simulink model "car_model"  (R2022b)
settings: Solver=VariableStepAuto  StartTime=0.0  StopTime=30  RelTol=1e-3
values from neighbouring files (symbols this model uses):
  X = Chassis_Signals.InertFrm.Cg.Disp.X.Data(:)    [Simulation_Data_Parse.m]    (also in Vehicle_Sim_Parse.m)
  Y = Chassis_Signals.InertFrm.Cg.Disp.Y.Data(:)    [Simulation_Data_Parse.m]    (also in Vehicle_Sim_Parse.m)
undefined symbols (not defined in the file or in its folder): ABS_MAX_TORQUE, ABS_MAX_TRQ_CMD, ABS_MIN_TORQUE, acc_IC, ACCELERATION_MAX, ActSuspDutyCycle, Aeq_left, Aeq_right, alpha_error, ang_acc_hystersesis, ang_IC, ang_vel_IC, area_air, axb, battery_current_IC, BATTERY_CURRENT_MAX, BATTERY_CURRENT_MIN, battery_FT_IC, battery_T_IC, BATTERY_TEMPERATURE_MAX, BATTERY_TEMPERATURE_MIN, battery_voltage_IC, BATTERY_VOLTAGE_MAX, BATTERY_VOLTAGE_MIN, Brake_Pressure_IC, ccl_IC, CENTER_STEER_ANGLE_MAX, covA, covarience_matrix_IC, covG, covM, covP, covV, cy_sweep, dB, dcl_IC, DCL_MAX, DCL_MIN, deadband_angle, dIndex, DiscIntNeverNeededParam, disk_abore, driver_t, dt_OFF, dt_ON, dTx, dx, dZ, F0z, forward_look_straight, forward_look_turn, fusion_t, fusion_t_sim, Fz_IC, Fz_sweep, g, gearbox_efficiency, gps_counter_IC, gps_ratio, gr ... (+105)
libraries: fl_lib x62, nesl_utility x16, vehdynlibtire x10, vehdynlibsuspension x8, simulink x5, autolibutils x5, sharedtransform x5, EngineCoolingComponents_lib x4, slpidlib x3, SimscapeFluids_lib x3, dspstat3 x2, shared6dof x2
(part 1 of 10)
settings Model: SimulationMode=accelerator  TunableVars=covA,covM,covP,covV,covG,phi,ref_location,ref_mag_field,location_lla_IC,gps_ratio,noise_state,fusion_t,ABS_MAX_TORQUE,MOTOR_ENABLE,BATTERY_CURRENT_MAX,deadband_angle,alpha_error,I,P,Torque_Up_Rate_Limit,Torque_Down_Rate_Limit,CURRENT_BUFFER,TVS_Intensity  TunableVarsStorageClass=Auto,Auto,Auto,Auto,Auto,Auto,Auto,Auto,Auto,Auto,Auto,Auto,Auto,Auto,Auto,Auto,Auto,Auto,Auto,Auto,Auto,Auto,Auto  TunableVarsTypeQualifier=,,,,,,,,,,,,,,,,,,,,,,  Creator=Inver  LastModifiedBy=Inver
settings DataIOCC: SaveFormat=StructureWithTime  SaveOutput=off  DSMLogging=off
settings OptimizationCC: DefaultParameterBehavior=Inlined  UseDivisionForNetSlopeComputation=on  GainParamInheritBuiltInType=on  UseFloatMulNetSlope=on  InlineInvariantSignals=on  PassReuseOutputArgsAs=Individual arguments  ZeroExternalMemoryAtStartup=off  ZeroInternalMemoryAtStartup=off  NoFixptDivByZeroProtection=on  EfficientFloat2IntCast=on  LifeSpan=1  OptimizeBlockOrder=speed  DifferentSizesBufferReuse=on  EfficientTunableParamExpr=on
settings DebuggingCC: ReadBeforeWriteMsg=DisableAll  WriteAfterWriteMsg=DisableAll  WriteAfterReadMsg=DisableAll  MultiTaskDSMMsg=none  ParameterTunabilityLossMsg=error  UnderSpecifiedDataTypeMsg=warning  UnderSpecifiedDimensionMsg=warning
settings HardwareCC: ProdBitPerPointer=32  ProdBitPerSizeT=32  ProdBitPerPtrDiffT=32  ProdLargestAtomicInteger=Long  ProdLargestAtomicFloat=Double  ProdWordSize=32  ProdLongLongMode=on  ProdHWDeviceType=ARM Compatible->ARM Cortex-M
settings ModelReferenceCC: EnableRefExpFcnMdlSchedulingChecks=on
settings SFSimCC: SimCustomHeaderCode="#include \"simplex.h\""  SimUserSources=C_Code/simplex.c  SFSimEcho=off  MATLABDynamicMemAlloc=off
settings RTWCC: Description=Embedded Coder  SystemTargetFile=ert.tlc  TemplateMakefile=ert_default_tmf  Toolchain=GNU Tools for ARM Embedded Processors
settings CodeAppCC: ForceParamTrailComments=on  IgnoreCustomStorageClasses=off  OperatorAnnotations=on  SimulinkDataObjDesc=on  SFDataObjDesc=on  CustomSymbolStrGlobalVar=rt$N$M  CustomSymbolStrType=$N$M  CustomSymbolStrFcn=$N$M$F  CustomSymbolStrMacro=$N$M  InsertBlockDesc=on
settings ERTTargetCC: TargetLangStandard=C99 (ISO)  GenerateSampleERTMain=on  IncludeMdlTerminateFcn=off  CombineSignalStateStructs=on  CodeInterfacePackaging=Reusable function  SupportComplex=off  SupportNonInlinedSFcns=on  InlinedParameterPlacement=NonHierarchical  RootIOFormat=Structure reference  ERTCustomFileTemplate=example_file_process.tlc  ERTFilePackagingFormat=CompactWithDataFile

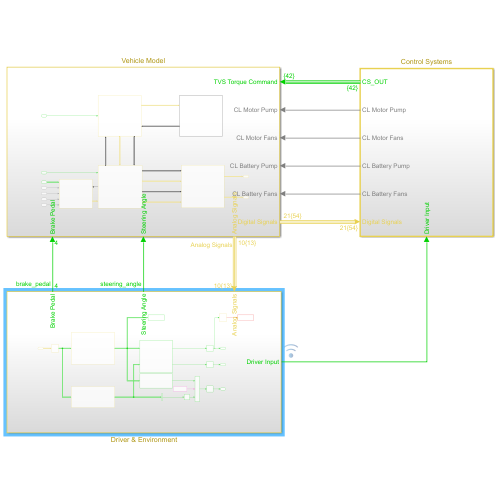
[thumbnail: Simulink's stored preview of the top-level diagram]
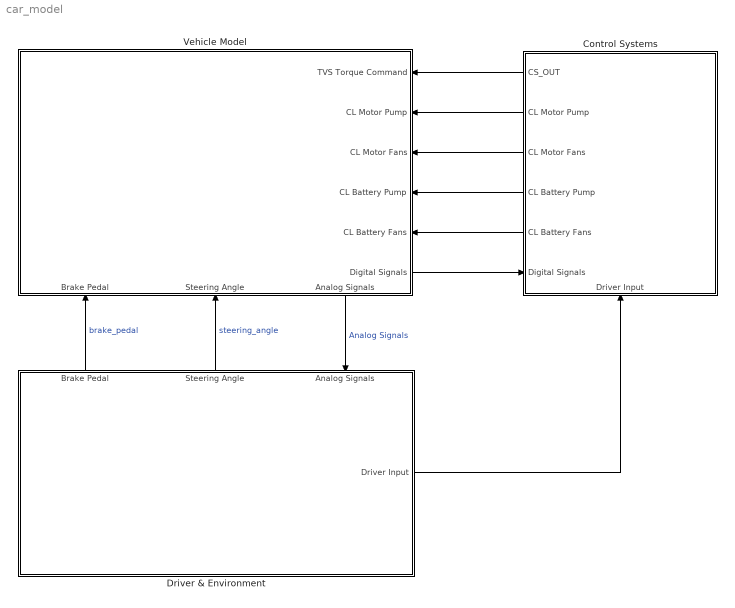
== system car_model ==
  Control Systems : Subsystem  TreatAsAtomicUnit=on  RTWFcnName=TVS_SYSTEM  RTWFileName=TVS_SYSTEM
      settings: PortSchema="{\"entries\":[{\"content\":{\"sides\":[{\"content\":{\"connectorIds\":[\"Out1\",\"Out2\",\"Out3\",\"Out4\",\"Out5\",\"In1\"]},\"type\":\"ConnectorPlacement.EquallySpacedRectSide\",\"uuid\":\"b5513b79-39cc-4156-8758-e9dd7d224c4f\"},{\"content\":{\"connectorIds\":[],\"side\":\"RIGHT\"},\"type\":\"ConnectorPlacement.EquallySpacedRectSide\",\"uuid\":\"18919d17-351d-4641-ab2c-66cbba916b4f\"},{\"content\":{\"connectorIds\":[],\"side\":\"TOP\"},\"type\":\"ConnectorPlacement.EquallySpacedRectSide\",\"uuid\":\"63240dfa-789e-427a-a529-4bce5e7f3f10\"},{\"content\":{\"connectorIds\":[\"In2\"],\"side\":\"BOTTOM\"},\"type\":\"ConnectorPlacement.EquallySpacedRectSide\",\"uuid\":\"43cc723f-5f4e-4e66-a14e-4ae2f3e16f9e\"}]},\"type\":\"ConnectorPlacement.EquallySpacedConnector\",\"uuid\":\"47be9ba7-cea3-4b3b-9ee6-e23e075e553b\"}],\"packageUris\":[\"http://schema.mathworks.com/mf0/Connector/R2020b\"],\"version\":\"1.0\"}"
  Driver & Environment : Subsystem
      settings: PortSchema="{\"entries\":[{\"content\":{\"sides\":[{\"content\":{\"connectorIds\":[]},\"type\":\"ConnectorPlacement.EquallySpacedRectSide\",\"uuid\":\"bd499254-800d-4f65-9d66-206e4f6126a9\"},{\"content\":{\"connectorIds\":[\"Out1\"],\"side\":\"RIGHT\"},\"type\":\"ConnectorPlacement.EquallySpacedRectSide\",\"uuid\":\"787bb70a-048d-46a8-9404-9c629bdce5fb\"},{\"content\":{\"connectorIds\":[\"Out2\",\"Out3\",\"In1\"],\"side\":\"TOP\"},\"type\":\"ConnectorPlacement.EquallySpacedRectSide\",\"uuid\":\"94a1f635-0878-46b0-949b-f2a3fa746134\"}]},\"type\":\"ConnectorPlacement.EquallySpacedConnector\",\"uuid\":\"f81a85a8-63b1-46ab-bae2-7f37115d6b57\"}],\"packageUris\":[\"http://schema.mathworks.com/mf0/Connector/R2020b\"],\"version\":\"1.0\"}"
  Vehicle Model : Subsystem
      settings: PortSchema="{\"entries\":[{\"content\":{\"sides\":[{\"content\":{\"connectorIds\":[]},\"type\":\"ConnectorPlacement.EquallySpacedRectSide\",\"uuid\":\"7263df3d-11c2-488e-998f-6bd776306b9c\"},{\"content\":{\"connectorIds\":[\"In3\",\"In4\",\"In5\",\"In6\",\"In7\",\"Out1\"],\"side\":\"RIGHT\"},\"type\":\"ConnectorPlacement.EquallySpacedRectSide\",\"uuid\":\"b0de89c2-35d2-4c59-81fc-f1f509ccf522\"},{\"content\":{\"connectorIds\":[],\"side\":\"TOP\"},\"type\":\"ConnectorPlacement.EquallySpacedRectSide\",\"uuid\":\"474ba072-8402-41d1-8015-97ca573757b9\"},{\"content\":{\"connectorIds\":[\"In1\",\"In2\",\"Out2\"],\"side\":\"BOTTOM\"},\"type\":\"ConnectorPlacement.EquallySpacedRectSide\",\"uuid\":\"2efad9e8-b0d8-4de5-bddc-0b63eaa22f81\"}]},\"type\":\"ConnectorPlacement.EquallySpacedConnector\",\"uuid\":\"426f55ca-7f3f-41f0-94e6-91e6d6304a5e\"}],\"packageUris\":[\"http://schema.mathworks.com/mf0/Connector/R2020b\"],\"version\":\"1.0\"}"
  wires:
  Control Systems/1(CS_OUT) -> Vehicle Model/3(TVS Torque Command)
  Driver & Environment/2(Brake Pedal) -> Vehicle Model/1(Brake Pedal)  "brake_pedal"
  Driver & Environment/3(Steering Angle) -> Vehicle Model/2(Steering Angle)  "steering_angle"
  Vehicle Model/2(Analog Signals) -> Driver & Environment/1(Analog Signals)  "Analog Signals"
  Vehicle Model/1(Digital Signals) -> Control Systems/1(Digital Signals)
  Driver & Environment/1(Driver Input) -> Control Systems/2(Driver Input)
  Control Systems/2(CL Motor Pump) -> Vehicle Model/4(CL Motor Pump)
  Control Systems/4(CL Battery Pump) -> Vehicle Model/6(CL Battery Pump)
  Control Systems/3(CL Motor Fans) -> Vehicle Model/5(CL Motor Fans)
  Control Systems/5(CL Battery Fans) -> Vehicle Model/7(CL Battery Fans)

== system car_model/Control Systems ==
  Digital Signals : Inport
  Driver Input : Inport  Port=2
  Bus Creator : BusCreator  Inputs=9
  Bus Selector : BusSelector  OutputSignals=Corner Dynamics Sensors.theta,Corner Dynamics Sensors.omega,Power Sensors.pwr_lmt,Power Sensors.motor_V,Power Sensors.motor_I,Power Sensors.batt_V,Power Sensors.batt_I,Cooling Sensors.motor_T,Cooling Sensors.mc_T
  Bus Selector1 : BusSelector  OutputSignals=Navigation Sensors.mag,Navigation Sensors.gyro,Navigation Sensors.acc,Navigation Sensors.pos,Navigation Sensors.vel
  Bus Selector2 : BusSelector  OutputSignals=angvel_VNED,vel_VNED
  Bus Selector3 : BusSelector  OutputSignals=Cooling Sensors.motor_T,Cooling Sensors.motor_FT,Cooling Sensors.batt_T,Cooling Sensors.batt_FT
  Bus Selector4 : BusSelector  OutputSignals=Corner Dynamics Sensors.shock_L,Corner Dynamics Sensors.FZ
  CLC : Subsystem
  NFE : Subsystem
  Sensor Fusion : Subsystem  TreatAsAtomicUnit=on  SystemSampleTime=fusion_t_sim
  TV Output Bus : BusCreator  Inputs=17
  TVS : Subsystem  TreatAsAtomicUnit=on  SystemSampleTime=tvs_t_sim
  To Workspace : ToWorkspace  VariableName=TV_Output  SaveFormat=Timeseries  SampleTime=-1
  To Workspace2 : ToWorkspace  VariableName=Sensor_Fused  SaveFormat=Timeseries  SampleTime=-1
  CS_OUT : Outport
  CL Motor Pump : Outport  Port=2
  CL Motor Fans : Outport  Port=3
  CL Battery Pump : Outport  Port=4
  CL Battery Fans : Outport  Port=5
  wires:
  Digital Signals/1 -> Bus Selector3/1, Bus Selector1/1, Bus Selector4/1, Bus Selector/1
  Bus Selector4/1 -> NFE/1(shock_L)  "<shock_L>"
  Bus Selector3/1 -> CLC/1(motor_temperature)  "<motor_T>"
  Bus Selector3/2 -> CLC/2(motor_fluid_temperature)  "<motor_FT>"
  Bus Selector3/3 -> CLC/3(battery_temperature)  "<batt_T>"
  Bus Selector3/4 -> CLC/4(battery_fluid_temperature)  "<batt_FT>"
  CLC/1(CL Motor Pump) -> CL Motor Pump/1
  CLC/2(CL Battery Pump) -> CL Battery Pump/1
  CLC/3(CL Motor Fans) -> CL Motor Fans/1
  CLC/4(CL Battery Fans) -> CL Battery Fans/1
  Bus Selector4/2 -> NFE/2(<Fz>)  "<FZ>"
  Bus Creator/1 -> To Workspace2/1, Bus Selector2/1
  Bus Selector1/1 -> Sensor Fusion/1(mag)  "<mag>"
  TV Output Bus/1 -> To Workspace/1, CS_OUT/1
  Driver Input/1 -> TVS/1(driver_input)
  NFE/1(Fz) -> TVS/11(Fz)
  Bus Selector2/1 -> TVS/12(angvel_VNED)  "<angvel_VNED>"
  Bus Selector1/2 -> Sensor Fusion/2(gyro)  "<gyro>"
  Bus Selector1/3 -> Sensor Fusion/3(accel)  "<acc>"
  Bus Selector1/4 -> Sensor Fusion/4(pos)  "<pos>"
  Bus Selector1/5 -> Sensor Fusion/5(vel)  "<vel>"
  Sensor Fusion/1(angvel_VNED) -> Bus Creator/1  "angvel_VNED"
  Sensor Fusion/2(ang_NED) -> Bus Creator/2  "ang_NED"
  Sensor Fusion/3(pos_VNED) -> Bus Creator/3  "pos_VNED"
  Sensor Fusion/4(vel_VNED) -> Bus Creator/4  "vel_VNED"
  Sensor Fusion/5(acc_VNED) -> Bus Creator/5  "acc_VNED"
  Sensor Fusion/6(mag_VNED) -> Bus Creator/6  "mag_VNED"
  Sensor Fusion/7(acc_bias_VNED) -> Bus Creator/7  "acc_bias_VNED"
  Sensor Fusion/8(gyro_bias_VNED) -> Bus Creator/8  "gyro_bias_VNED"
  Sensor Fusion/9(mag_bias_VNED) -> Bus Creator/9  "mag_bias_VNED"
  TVS/1(ref_yaw) -> TV Output Bus/1  "ref_yaw"
  TVS/2(beq) -> TV Output Bus/2  "beq"
  TVS/3(obj_gain) -> TV Output Bus/3  "obj_gain"
  TVS/4(lb) -> TV Output Bus/4  "lb"
  TVS/5(ub) -> TV Output Bus/5  "ub"
  TVS/6(windup) -> TV Output Bus/6  "windup"
  TVS/7(Aeq) -> TV Output Bus/7  "Aeq"
  TVS/8(b) -> TV Output Bus/8  "b"
  TVS/9(Tx) -> TV Output Bus/9  "Tx"
  TVS/10(bigM_flag) -> TV Output Bus/10  "bigM_flag"
  TVS/11(omega_m_TV) -> TV Output Bus/11  "omega_m"
  TVS/12(max_ang_acc) -> TV Output Bus/12  "max_ang_acc"
  TVS/13(min_ang_acc) -> TV Output Bus/13  "min_ang_acc"
  TVS/14(motor_I) -> TV Output Bus/14  "motor_I"
  TVS/15(motor_V) -> TV Output Bus/15  "motor_V"
  TVS/16(I_limits) -> TV Output Bus/16  "current_limits"
  TVS/17(batt_V) -> TV Output Bus/17  "battery_V"
  Bus Selector2/2 -> TVS/13(vel_VNED)  "<vel_VNED>"
  Bus Selector/1 -> TVS/2(steering_angle)  "<theta>"
  Bus Selector/2 -> TVS/3(omega)  "<omega>"
  Bus Selector/3 -> TVS/4(current_limits)  "<pwr_lmt>"
  Bus Selector/4 -> TVS/5(motor_voltage)  "<motor_V>"
  Bus Selector/5 -> TVS/6(motor_current)  "<motor_I>"
  Bus Selector/6 -> TVS/7(battery_voltage)  "<batt_V>"
  Bus Selector/7 -> TVS/8(battery_current)  "<batt_I>"
  Bus Selector/8 -> TVS/9(motor_temp)  "<motor_T>"
  Bus Selector/9 -> TVS/10(mc_temp)  "<mc_T>"

== system car_model/Driver & Environment ==
  Analog Signals : Inport
  Bus Selector : BusSelector  OutputSignals=Steering Angle
  Bus Selector1 : BusSelector  OutputSignals=GndFz
  Constant : Constant  Value=YAW_ENABLE
  Lateral Control : Subsystem
  Longitudinal Control : Subsystem
      settings: PortSchema="{\"entries\":[{\"content\":{\"sides\":[{\"content\":{\"connectorIds\":[\"In1\",\"In2\",\"In3\"]},\"type\":\"ConnectorPlacement.EquallySpacedRectSide\",\"uuid\":\"c84d1b45-47cb-44c3-9bb8-057964d890de\"},{\"content\":{\"connectorIds\":[\"Out1\",\"Out2\",\"In4\"],\"side\":\"RIGHT\"},\"type\":\"ConnectorPlacement.EquallySpacedRectSide\",\"uuid\":\"136455d0-d36a-4818-af11-72b5a1b8c27c\"},{\"content\":{\"connectorIds\":[],\"side\":\"TOP\"},\"type\":\"ConnectorPlacement.EquallySpacedRectSide\",\"uuid\":\"42b2ce8c-2720-4fbc-908c-f7068b304798\"}]},\"type\":\"ConnectorPlacement.EquallySpacedConnector\",\"uuid\":\"ec27d525-5c9d-4748-8b13-bb528198656f\"}],\"packageUris\":[\"http://schema.mathworks.com/mf0/Connector/R2020b\"],\"version\":\"1.0\"}"
  Rate Limiter : RateLimiter  RisingSlewLimit=MAX_DTHETA_DRIVER  FallingSlewLimit=-MAX_DTHETA_DRIVER  SampleTimeMode=inherited
  Rate Transition : RateTransition  OutPortSampleTime=driver_t
  Reference Generator : Subsystem
  Sweep Generator : Subsystem
  Switch : Switch  Criteria=u2 > Threshold  SaturateOnIntegerOverflow=off  InputSameDT=off
  To Workspace1 : ToWorkspace  VariableName=Throttle  SaveFormat=Timeseries  SampleTime=-1
  Unit Delay : UnitDelay  InitialCondition=Brake_Pressure_IC  SampleTime=driver_t  HasFrameUpgradeWarning=on
  Unit Delay1 : UnitDelay  SampleTime=driver_t  HasFrameUpgradeWarning=on
  Unit Delay2 : UnitDelay  SampleTime=driver_t  HasFrameUpgradeWarning=on
  Driver Input : Outport
  Brake Pedal : Outport  Port=2
  Steering Angle : Outport  Port=3
  wires:
  Longitudinal Control/2(brake_pedal) -> Unit Delay/1  "brake_pressure_pa"
  Lateral Control/1(steering_angle) -> Switch/1  "center_column_steering_angle_deg"
  Longitudinal Control/1(driver_input) -> Unit Delay2/1  "driver_input"
  Switch/1 -> Unit Delay1/1
  Analog Signals/1 -> Rate Transition/1
  Constant/1 -> Switch/2
  Rate Limiter/1 -> Switch/3
  Rate Transition/1 -> Bus Selector1/1, Sweep Generator/1(Analog Signals), Reference Generator/1(Analog Signals)
  Unit Delay1/1 -> Steering Angle/1, Longitudinal Control/4(In3)
  Unit Delay/1 -> Brake Pedal/1
  Reference Generator/1(Controller Information) -> Lateral Control/1(Controller Information), Longitudinal Control/1(Controller Information)
  Sweep Generator/1(Controller Information) -> Longitudinal Control/3(Sweep Information), Bus Selector/1
  Bus Selector/1 -> Rate Limiter/1  "<Steering Angle>"
  Unit Delay2/1 -> Driver Input/1, To Workspace1/1  "throttle"
  Bus Selector1/1 -> Longitudinal Control/2(In2)  "<GndFz>"

== system car_model/Vehicle Model ==
  Brake Pedal : Inport
  Steering Angle : Inport  Port=2
  TVS Torque Command : Inport  Port=3
  CL Motor Pump : Inport  Port=4
  CL Motor Fans : Inport  Port=5
  CL Battery Pump : Inport  Port=6
  CL Battery Fans : Inport  Port=7
  Electronics : Subsystem
  Powertrain : Subsystem
      settings: PortSchema="{\"entries\":[{\"content\":{\"sides\":[{\"content\":{\"connectorIds\":[\"In1\",\"In2\",\"In3\",\"In4\",\"In5\"]},\"type\":\"ConnectorPlacement.EquallySpacedRectSide\",\"uuid\":\"895a90fc-946f-4344-af69-c005acf2f614\"},{\"content\":{\"connectorIds\":[\"In6\",\"Out1\"],\"side\":\"RIGHT\"},\"type\":\"ConnectorPlacement.EquallySpacedRectSide\",\"uuid\":\"931fcb49-b75e-480c-a4d6-2f82b080d057\"},{\"content\":{\"connectorIds\":[],\"side\":\"TOP\"},\"type\":\"ConnectorPlacement.EquallySpacedRectSide\",\"uuid\":\"d1b12b51-387e-4553-b5da-149d57232505\"}]},\"type\":\"ConnectorPlacement.EquallySpacedConnector\",\"uuid\":\"0cb2c3dd-4627-421c-9ed4-7e8c572a9937\"}],\"packageUris\":[\"http://schema.mathworks.com/mf0/Connector/R2020b\"],\"version\":\"1.0\"}"
  Suspension : Subsystem  Variant=on  VariantControlMode=label  LabelModeActiveChoice=1
      settings: PortSchema="{\"entries\":[{\"content\":{\"sides\":[{\"content\":{\"connectorIds\":[\"In1\"]},\"type\":\"ConnectorPlacement.EquallySpacedRectSide\",\"uuid\":\"d90bf910-501d-4dd1-a367-d76bd42ab174\"},{\"content\":{\"connectorIds\":[\"Out1\",\"In3\"],\"side\":\"RIGHT\"},\"type\":\"ConnectorPlacement.EquallySpacedRectSide\",\"uuid\":\"1fe7da07-1086-4d5e-8baf-d5d069455d6e\"},{\"content\":{\"connectorIds\":[],\"side\":\"TOP\"},\"type\":\"ConnectorPlacement.EquallySpacedRectSide\",\"uuid\":\"6ff63b9e-45bb-47e9-90cd-47f8e0815e57\"},{\"content\":{\"connectorIds\":[\"In2\",\"Out2\",\"Out3\"],\"side\":\"BOTTOM\"},\"type\":\"ConnectorPlacement.EquallySpacedRectSide\",\"uuid\":\"116c6de0-7bfa-4dc1-bfd0-57a2fffb3aa0\"}]},\"type\":\"ConnectorPlacement.EquallySpacedConnector\",\"uuid\":\"6475b998-12b0-4b0e-8a20-c379b8e08c7c\"}],\"packageUris\":[\"http://schema.mathworks.com/mf0/Connector/R2020b\"],\"version\":\"1.0\"}"
      mask Display:
      | switch str2num(get_param(gcb,'ActiveVariant'))
      |     case 1
      |         image('suspdw.png');
      |     case 2
      |         image([imread('suspindmap.png');imread('suspsamap.png')]);
      |     case 3
      |          image([imread('suspmacp.png');imread('suspsacoil.png')]);
      |     case 4
      |          image('suspmacp.png');
      |     case 5
      |          image('suspindmap.png');
      |     case 6
      |          image('suspkandc.png');
      | end
  Vehicle : Subsystem
      settings: PortSchema="{\"entries\":[{\"content\":{\"sides\":[{\"content\":{\"connectorIds\":[\"In1\",\"Out1\"]},\"type\":\"ConnectorPlacement.EquallySpacedRectSide\",\"uuid\":\"63fa377f-0583-4c60-bac7-9bd73dadd9a1\"},{\"content\":{\"connectorIds\":[],\"side\":\"RIGHT\"},\"type\":\"ConnectorPlacement.EquallySpacedRectSide\",\"uuid\":\"7f668e34-aa5e-4f2f-9be8-80fbb83ff2c8\"},{\"content\":{\"connectorIds\":[],\"side\":\"TOP\"},\"type\":\"ConnectorPlacement.EquallySpacedRectSide\",\"uuid\":\"511f439c-568f-45f1-9ff4-54e644eb8180\"}]},\"type\":\"ConnectorPlacement.EquallySpacedConnector\",\"uuid\":\"b54bf87e-fa06-468b-8fa9-38148d60ed3d\"}],\"packageUris\":[\"http://schema.mathworks.com/mf0/Connector/R2020b\"],\"version\":\"1.0\"}"
      mask Display: image('6dofcar.png');
  Wheels and Tires : Subsystem
      settings: PortSchema="{\"entries\":[{\"content\":{\"sides\":[{\"content\":{\"connectorIds\":[\"In1\",\"Out6\",\"In2\"]},\"type\":\"ConnectorPlacement.EquallySpacedRectSide\",\"uuid\":\"77263124-783e-4307-b979-a6212540af24\"},{\"content\":{\"connectorIds\":[\"Out1\",\"Out2\",\"Out3\",\"Out4\"],\"side\":\"RIGHT\"},\"type\":\"ConnectorPlacement.EquallySpacedRectSide\",\"uuid\":\"cb03b446-69c2-4dbf-929b-d33818acfe8b\"},{\"content\":{\"connectorIds\":[\"Out5\",\"In3\",\"In4\"],\"side\":\"TOP\"},\"type\":\"ConnectorPlacement.EquallySpacedRectSide\",\"uuid\":\"8e7e4023-62e5-48a8-8666-b4c8bb14cd01\"}]},\"type\":\"ConnectorPlacement.EquallySpacedConnector\",\"uuid\":\"1061f0db-ec8e-49bd-8d66-b4a53eaeacfa\"}],\"packageUris\":[\"http://schema.mathworks.com/mf0/Connector/R2020b\"],\"version\":\"1.0\"}"
      mask Display: image('wheel3dof.png')
  Digital Signals : Outport  PortDimensions={292}
  Analog Signals : Outport  Port=2  PortDimensions={292}
  wires:
  Steering Angle/1 -> Suspension/1(Steering)
  Suspension/1(Suspension) -> Vehicle/1(Suspension)  "Susp"
  Wheels and Tires/5(Wheels2Susp) -> Suspension/2(Wheel)
  Powertrain/1(PwrTrn) -> Wheels and Tires/2(PwrTrn)
  Brake Pedal/1 -> Wheels and Tires/1(Brake Press)
  TVS Torque Command/1 -> Powertrain/1(TVS Torque Command)
  Suspension/2(Suspension1) -> Wheels and Tires/3(Sus)
  Vehicle/1(VehFdbk) -> Suspension/3(Vehicle)  "Vehicle"
  Suspension/3(Veh) -> Wheels and Tires/4(Veh)
  Wheels and Tires/1(Vehicle) -> Electronics/1(Veh)  "veh"
  Wheels and Tires/2(Suspension) -> Electronics/2(Sus)  "sus"
  Wheels and Tires/3(Wheels) -> Electronics/3(Whl)  "whl"
  Electronics/1(Analog Signals) -> Analog Signals/1
  Electronics/2(Digital Signals) -> Digital Signals/1
  Wheels and Tires/4(Power Train) -> Electronics/4(Trn)  "trn"
  CL Motor Pump/1 -> Powertrain/2(CL Motor Pump)
  CL Battery Pump/1 -> Powertrain/4(CL Battery Pump)
  CL Motor Fans/1 -> Powertrain/3(CL Motor Fans)
  CL Battery Fans/1 -> Powertrain/5(CL Battery Fans)
  Wheels and Tires/6(Vg) -> Powertrain/6(Vg)

== system car_model/Control Systems/CLC ==
  motor_temperature : Inport
  motor_fluid_temperature : Inport  Port=2
  battery_temperature : Inport  Port=3
  battery_fluid_temperature : Inport  Port=4
  Step : Step  After=0  SampleTime=0
  CL Motor Pump : Outport
  CL Battery Pump : Outport  Port=2
  CL Motor Fans : Outport  Port=3
  CL Battery Fans : Outport  Port=4
  wires:
  Step/1 -> CL Motor Fans/1, CL Battery Fans/1, CL Battery Pump/1, CL Motor Pump/1

== system car_model/Control Systems/NFE ==
  shock_L : Inport
  <Fz> : Inport  Port=2
  Saturation17 : Saturate  UpperLimit=1200  LowerLimit=200
  Terminator : Terminator
  Fz : Outport
  wires:
  shock_L/1 -> Terminator/1
  <Fz>/1 -> Saturation17/1
  Saturation17/1 -> Fz/1  "FZ"

== system car_model/Control Systems/Sensor Fusion ==
  mag : Inport
  gyro : Inport  Port=2
  accel : Inport  Port=3
  pos : Inport  Port=4
  vel : Inport  Port=5
  NED2VNED : MATLAB Function  TreatAsAtomicUnit=on
  SNED to VNED : MATLAB Function  TreatAsAtomicUnit=on
  Transpose{,1..11} (12 alike) : Math  Operator=transpose
  Unit Delay1 : UnitDelay  InitialCondition=gps_counter_IC  SampleTime=-1  HasFrameUpgradeWarning=on
  Unit Delay2 : UnitDelay  InitialCondition=state_IC  SampleTime=-1  HasFrameUpgradeWarning=on
  Unit Delay3 : UnitDelay  InitialCondition=covarience_matrix_IC  SampleTime=-1  HasFrameUpgradeWarning=on
  fusion : MATLAB Function  TreatAsAtomicUnit=on
  angvel_VNED : Outport
  ang_NED : Outport  Port=2
  pos_VNED : Outport  Port=3
  vel_VNED : Outport  Port=4
  acc_VNED : Outport  Port=5
  mag_VNED : Outport  Port=6
  acc_bias_VNED : Outport  Port=7
  gyro_bias_VNED : Outport  Port=8
  mag_bias_VNED : Outport  Port=9
  wires:
  NED2VNED/7(accel_bias) -> Transpose8/1  "acc_bias_VNED"
  NED2VNED/3(pos) -> Transpose9/1  "pos_VNED"
  NED2VNED/4(vel) -> Transpose5/1  "vel_VNED"
  NED2VNED/2(angvel) -> Transpose10/1  "angvel_VNED"
  NED2VNED/1(ang) -> Transpose11/1  "ang_NED"
  fusion/2(rot_map) -> NED2VNED/1(rot_map)
  Transpose/1 -> fusion/4(acceleration)
  Unit Delay3/1 -> fusion/8(cov_in)
  NED2VNED/8(gyro_bias) -> Transpose4/1  "gyro_bias_VNED"
  Transpose1/1 -> fusion/5(angularVelocity)
  fusion/4(cov_out) -> Unit Delay3/1
  fusion/3(state_out) -> Unit Delay2/1, NED2VNED/2(state)
  SNED to VNED/2(gyro_VNED) -> Transpose1/1  "gyro_VNED"
  SNED to VNED/1(accel_VNED) -> Transpose/1  "accel_VNED"
  NED2VNED/5(accel) -> Transpose6/1  "acc_VNED"
  SNED to VNED/3(mag_VNED) -> Transpose2/1  "mag_VNED"
  Unit Delay2/1 -> fusion/7(state_in)
  Transpose2/1 -> fusion/6(magField)
  NED2VNED/9(mag_bias) -> Transpose3/1  "mag_bias_VNED"
  NED2VNED/6(mag) -> Transpose7/1  "mag_VNED"
  accel/1 -> SNED to VNED/1(accel_SNED)
  gyro/1 -> SNED to VNED/2(gyro_SNED)
  mag/1 -> SNED to VNED/3(mag_SNED)
  pos/1 -> fusion/3(position)
  vel/1 -> fusion/2(velocity)
  Transpose3/1 -> mag_bias_VNED/1
  Transpose4/1 -> gyro_bias_VNED/1
  Transpose8/1 -> acc_bias_VNED/1
  Transpose7/1 -> mag_VNED/1
  Transpose6/1 -> acc_VNED/1
  Transpose5/1 -> vel_VNED/1
  Transpose9/1 -> pos_VNED/1
  Transpose10/1 -> angvel_VNED/1
  Transpose11/1 -> ang_NED/1
  fusion/1(count) -> Unit Delay1/1
  Unit Delay1/1 -> fusion/1("count ")

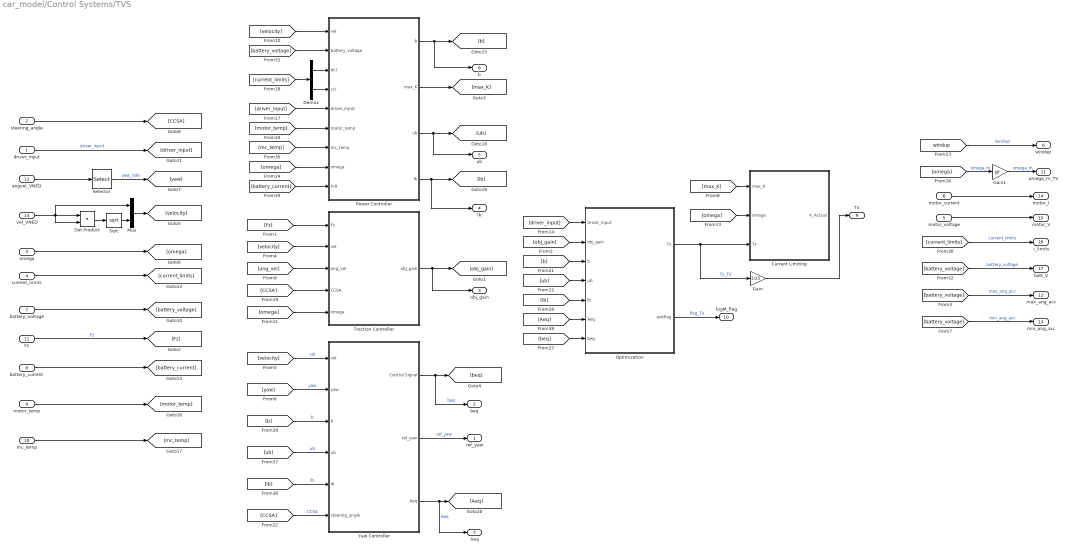
== system car_model/Control Systems/TVS ==
  driver_input : Inport  OutMin=-1  OutMax=1  OutDataTypeStr=double  PortDimensions=1  LockScale=on
  steering_angle : Inport  Port=2  OutMin=-130  OutMax=130  OutDataTypeStr=double  PortDimensions=1
  omega : Inport  Port=3  OutMin=0  OutMax=150  OutDataTypeStr=double  LockScale=on
  current_limits : Inport  Port=4  OutMin=-80000  OutMax=80000  OutDataTypeStr=double  LockScale=on
  motor_voltage : Inport  Port=5
  motor_current : Inport  Port=6
  battery_voltage : Inport  Port=7  OutMin=50  OutMax=340  OutDataTypeStr=double
  battery_current : Inport  Port=8
  motor_temp : Inport  Port=9
  mc_temp : Inport  Port=10
  Fz : Inport  Port=11
  angvel_VNED : Inport  Port=12  OutMin=-5  OutMax=5  OutDataTypeStr=double  PortDimensions=[1 3]  LockScale=on
  vel_VNED : Inport  Port=13  OutMin=0  OutMax=30  OutDataTypeStr=double  LockScale=on
  Current Limiting : Subsystem
  Demux : Demux  Outputs=2
  Dot Product : DotProduct  OutDataTypeStr=Inherit: Inherit via internal rule
  Gain : Gain  Gain=1/25
  Gain1 : Gain  Gain=gr  ParamDataTypeStr=double  OutDataTypeStr=Inherit: Inherit via back propagation
  Mux : Mux  Inputs=2
  Optimization : Subsystem
  Power Controller : Subsystem
  Selector : Selector  InputPortWidth=3  IndexOptions=Index vector (dialog)  Indices=3  OutputSizes=1
  Sqrt : Sqrt
  Traction Controller : Subsystem
  Yaw Controller : Subsystem
  ref_yaw : Outport
  beq : Outport  Port=2  OutMin=-10  OutMax=10  OutDataTypeStr=double  LockScale=on
  obj_gain : Outport  Port=3
  lb : Outport  Port=4  OutMin=-25  OutMax=25  OutDataTypeStr=double  LockScale=on
  ub : Outport  Port=5  OutMin=-25  OutMax=25  OutDataTypeStr=double  LockScale=on
  windup : Outport  Port=6
  Aeq : Outport  Port=7  OutMin=-1.9  OutMax=1.9  OutDataTypeStr=double  LockScale=on
  b : Outport  Port=8  OutMin=-80000  OutMax=80000  OutDataTypeStr=double  LockScale=on
  Tx : Outport  Port=9  OutDataTypeStr=double  PortDimensions=[1 4]
  bigM_flag : Outport  Port=10  PortDimensions=1
  omega_m_TV : Outport  Port=11
  max_ang_acc : Outport  Port=12
  min_ang_acc : Outport  Port=13
  motor_I : Outport  Port=14
  motor_V : Outport  Port=15
  I_limits : Outport  Port=16
  batt_V : Outport  Port=17
  wires:
  motor_current/1 -> motor_I/1
  motor_voltage/1 -> motor_V/1
  omega/1 -> [omega]
  [velocity] -> Traction Controller/2(vel)
  current_limits/1 -> [current_limits]
  Optimization/2(exitflag) -> bigM_flag/1  "flag_TV"
  vel_VNED/1 -> Mux/1, Dot Product/2, Dot Product/1
  [omega] -> Gain1/1  "omega_m"
  [velocity] -> Yaw Controller/1(vel)  "vel"
  [ang_vel] -> Traction Controller/3(ang_vel)
  Power Controller/1(b) -> b/1, [b]
  Traction Controller/1(obj_gain) -> [obj_gain], obj_gain/1
  Power Controller/3(ub) -> ub/1, [ub]
  angvel_VNED/1 -> Selector/1
  [omega] -> Traction Controller/5(omega)
  battery_voltage/1 -> [battery_voltage]
  [driver_input] -> Optimization/1(driver_input)
  Yaw Controller/1(Control Signal) -> [beq], beq/1  "beq"
  [yaw] -> Yaw Controller/2(yaw)  "yaw"
  [Fz] -> Traction Controller/1(Fz)
  [windup] -> windup/1  "windup"
  Yaw Controller/3(Aeq) -> [Aeq], Aeq/1  "Aeq"
  driver_input/1 -> [driver_input]  "driver_input"
  [beq] -> Optimization/7(beq)
  Power Controller/4(lb) -> lb/1, [lb]
  Fz/1 -> [Fz]  "Fz"
  [obj_gain] -> Optimization/2(obj_gain)
  Yaw Controller/2(ref_yaw) -> ref_yaw/1  "ref_yaw"
  [current_limits] -> I_limits/1  "current_limits"
  [battery_voltage] -> batt_V/1  "battery_voltage"
  battery_current/1 -> [battery_current]
  Selector/1 -> [yaw]  "yaw_rate"
  Dot Product/1 -> Sqrt/1
  Mux/1 -> [velocity]
  Sqrt/1 -> Mux/2
  motor_temp/1 -> [motor_temp]
  mc_temp/1 -> [mc_temp]
  Gain1/1 -> omega_m_TV/1  "omega_m"
  steering_angle/1 -> [CCSA]
  [CCSA] -> Traction Controller/4(CCSA)
  [velocity] -> Power Controller/1(vel)
  [battery_voltage] -> Power Controller/2(battery_voltage)
  [battery_current] -> Power Controller/9(In9)
  [driver_input] -> Power Controller/5(driver_input)
  [motor_temp] -> Power Controller/6(motor_temp)
  [mc_temp] -> Power Controller/7(mc_temp)
  [current_limits] -> Demux/1
  Demux/2 -> Power Controller/4(ccl)
  Demux/1 -> Power Controller/3(dcl)
  [CCSA] -> Yaw Controller/6(steering_angle)  "CCSA"
  [ub] -> Optimization/4(ub)
  [lb] -> Optimization/5(lb)
  [b] -> Optimization/3(b)
  [ub] -> Yaw Controller/4(ub)  "ub"
  [lb] -> Yaw Controller/5(lb)  "lb"
  [b] -> Yaw Controller/3(b)  "b"
  [Aeq] -> Optimization/6(Aeq)
  [omega] -> Power Controller/8(omega)
  [battery_voltage] -> max_ang_acc/1  "max_ang_acc"
  [battery_voltage] -> min_ang_acc/1  "min_ang_acc"
  [max_K] -> Current Limiting/1(max_K)
  Power Controller/2(max_K) -> [max_K]
  [omega] -> Current Limiting/2(omega)
  Optimization/1(Tx) -> Gain/1, Current Limiting/3(Tx)  "Tx_TV"
  Gain/1 -> Tx/1

== system car_model/Driver & Environment/Lateral Control ==
  Controller Information : Inport
  1-D Lookup Table : Lookup_n-D  NumberOfTableDimensions=1  BreakpointsForDimension1=velocity_sweep  Table=max_yaw  ExtrapMethod=Clip  InternalRulePriority=Speed  RndMeth=Simplest
  2-D Lookup Table1 : Lookup_n-D  BreakpointsForDimension1=yaw_rate_sweep  BreakpointsForDimension2=velocity_sweep  Table=steering_Up_Grid  ExtrapMethod=Clip  InternalRulePriority=Speed  RndMeth=Simplest
      settings: InputPortMap=u0,u1
  2-D Lookup Table2 : Lookup_n-D  BreakpointsForDimension1=yaw_rate_sweep  BreakpointsForDimension2=velocity_sweep  Table=steering_Up_Grid  ExtrapMethod=Clip  InternalRulePriority=Speed  RndMeth=Simplest
      settings: InputPortMap=u0,u1
  Abs : Abs  SaturateOnIntegerOverflow=off
  Bus Selector : BusSelector  OutputSignals=p_error,Vnow,yaw_ref,v_cog
  Constant : Constant  Value=17.5
  Constant1 : Constant  Value=0
  GreaterThan : RelationalOperator  Operator=>  OutDataTypeStr=boolean  RndMeth=Simplest  InputSameDT=off
  GreaterThan1 : RelationalOperator  Operator=~=  OutDataTypeStr=boolean  RndMeth=Simplest  InputSameDT=off
  Min : MinMax  Inputs=2
  NAND : Logic  Operator=NAND  IconShape=distinctive  AllPortsSameDT=off  OutDataTypeStr=boolean
  NOT : Logic  Operator=NOT  IconShape=distinctive  AllPortsSameDT=off  OutDataTypeStr=boolean
  PID Controller : slpidlib/PID Controller  Controller=PID  Form=Parallel  TimeDomain=Discrete-time  UseExternalTs=off  SampleTime=-1  IntegratorMethod=Forward Euler  FilterMethod=Forward Euler  ControllerParametersSource=internal  P=P_Straight_Adjust  I=0  UseKiTs=on  D=0  N=0  UseFilter=on  TunerSelectOption=Transfer Function Based (PID Tuner App)  InitialConditionSource=internal  InitialConditionForIntegrator=0  InitialConditionForFilter=0  DifferentiatorICPrevScaledInput=0  ExternalReset=none  TrackingMode=off  Kt=1  LimitOutput=on  SatLimitsSource=internal  UpperSaturationLimit=MAX_STEERING_ADJUST  LowerSaturationLimit=-MAX_STEERING_ADJUST  LinearizeAsGain=on  AntiWindupMode=none  Kb=1  LimitIntegrator=off  UpperIntegratorSaturationLimit=inf  LowerIntegratorSaturationLimit=-inf  POutMin=[]  POutMax=[]  IOutMin=[]  IOutMax=[]  DOutMin=[]  DOutMax=[]  NOutMin=[]  NOutMax=[]  SumOutMin=[]  SumOutMax=[]  SaturationOutMin=[]  SaturationOutMax=[]  PParamMin=[]  PParamMax=[]  IParamMin=[]  IParamMax=[]  DParamMin=[]  DParamMax=[]  NParamMin=[]  NParamMax=[]  KbParamMin=[]  KbParamMax=[]  KtParamMin=[]  KtParamMax=[]  KbOutMin=[]  KbOutMax=[]  KtOutMin=[]  KtOutMax=[]  IntegratorOutMin=[]  IntegratorOutMax=[]  FilterOutMin=[]  FilterOutMax=[]  SumI1OutMin=[]  SumI1OutMax=[]  SumI2OutMin=[]  SumI2OutMax=[]  SumI3OutMin=[]  SumI3OutMax=[]  SumI4OutMin=[]  SumI4OutMax=[]  SumDOutMin=[]  SumDOutMax=[]  DifferentiatorOutMin=[]  DifferentiatorOutMax=[]  FilterDiffOutCoefMin=[]  FilterDiffOutCoefMax=[]  ReciprocalOutMin=[]  ReciprocalOutMax=[]  SumDenOutMin=[]  SumDenOutMax=[]  SumNumOutMin=[]  SumNumOutMax=[]  DivideOutMin=[]  DivideOutMax=[]  UdiffTsProdOutMin=[]  UdiffTsProdOutMax=[]  NTsProdOutMin=[]  NTsProdOutMax=[]  UintegralTsProdOutMin=[]  UintegralTsProdOutMax=[]  UngainTsProdOutMin=[]  UngainTsProdOutMax=[]  ClampingZeroOutDataTypeStr=Inherit: Inherit via back propagation  ClampingZeroOutMin=[]  ClampingZeroOutMax=[]  FilterDenConstantOutDataTypeStr=Inherit: Inherit via back propagation  FilterDenConstantOutMin=[]  FilterDenConstantOutMax=[]  PCopyOutDataTypeStr=Inherit: Inherit via back propagation  PCopyOutMin=[]  PCopyOutMax=[]  NCopyOutDataTypeStr=Inherit: Inherit via back propagation  NCopyOutMin=[]  NCopyOutMax=[]  IntegratorContinuousStateAttributes=''  IntegratorStateMustResolveToSignalObject=off  IntegratorRTWStateStorageClass=Auto  FilterContinuousStateAttributes=''  FilterStateMustResolveToSignalObject=off  FilterRTWStateStorageClass=Auto  ParallelPVariant=InternalParameters  IdealPVariant=Disabled  IVariant=InternalParameters  DVariant=InternalParameters  IntegratorVariant=Discrete  SatVariant=Enabled  AWVariant=Passthrough  PCopyVariant=Disabled  TRVariant=Disabled  FdbkBlocksVariant=Forward  IdealPFdbkVariant=Disabled  SatFdbkVariant=Disabled  DerivativeFilterVariant=ForwardEulerFilter  NVariant=InternalParameters  NCopyVariant=Disabled  FilterICVariant=InternalICsFilter  IntegratorICVariant=InternalICs  ExternalResetVariant=Disabled  TRSumVariant=Passthrough  SumFdbkVariant=Disabled  SumVariant=Sum_PID  TsampFilterVariant=InternalTs  TsampNgainVariant=Passthrough  TsampIntegralVariant=Passthrough  ExternalSaturationOutDataTypeStr=Inherit: Same as second input
  PID Controller1 : slpidlib/PID Controller  Controller=PID  Form=Parallel  TimeDomain=Discrete-time  UseExternalTs=off  SampleTime=-1  IntegratorMethod=Forward Euler  FilterMethod=Forward Euler  ControllerParametersSource=internal  P=P_Steering_Adjust  I=0  UseKiTs=on  D=0  N=0  UseFilter=on  TunerSelectOption=Transfer Function Based (PID Tuner App)  InitialConditionSource=internal  InitialConditionForIntegrator=0  InitialConditionForFilter=0  DifferentiatorICPrevScaledInput=0  ExternalReset=none  TrackingMode=off  Kt=1  LimitOutput=on  SatLimitsSource=internal  UpperSaturationLimit=MAX_STEERING_ADJUST  LowerSaturationLimit=-MAX_STEERING_ADJUST  LinearizeAsGain=on  AntiWindupMode=none  Kb=1  LimitIntegrator=off  UpperIntegratorSaturationLimit=inf  LowerIntegratorSaturationLimit=-inf  POutMin=[]  POutMax=[]  IOutMin=[]  IOutMax=[]  DOutMin=[]  DOutMax=[]  NOutMin=[]  NOutMax=[]  SumOutMin=[]  SumOutMax=[]  SaturationOutMin=[]  SaturationOutMax=[]  PParamMin=[]  PParamMax=[]  IParamMin=[]  IParamMax=[]  DParamMin=[]  DParamMax=[]  NParamMin=[]  NParamMax=[]  KbParamMin=[]  KbParamMax=[]  KtParamMin=[]  KtParamMax=[]  KbOutMin=[]  KbOutMax=[]  KtOutMin=[]  KtOutMax=[]  IntegratorOutMin=[]  IntegratorOutMax=[]  FilterOutMin=[]  FilterOutMax=[]  SumI1OutMin=[]  SumI1OutMax=[]  SumI2OutMin=[]  SumI2OutMax=[]  SumI3OutMin=[]  SumI3OutMax=[]  SumI4OutMin=[]  SumI4OutMax=[]  SumDOutMin=[]  SumDOutMax=[]  DifferentiatorOutMin=[]  DifferentiatorOutMax=[]  FilterDiffOutCoefMin=[]  FilterDiffOutCoefMax=[]  ReciprocalOutMin=[]  ReciprocalOutMax=[]  SumDenOutMin=[]  SumDenOutMax=[]  SumNumOutMin=[]  SumNumOutMax=[]  DivideOutMin=[]  DivideOutMax=[]  UdiffTsProdOutMin=[]  UdiffTsProdOutMax=[]  NTsProdOutMin=[]  NTsProdOutMax=[]  UintegralTsProdOutMin=[]  UintegralTsProdOutMax=[]  UngainTsProdOutMin=[]  UngainTsProdOutMax=[]  ClampingZeroOutDataTypeStr=Inherit: Inherit via back propagation  ClampingZeroOutMin=[]  ClampingZeroOutMax=[]  FilterDenConstantOutDataTypeStr=Inherit: Inherit via back propagation  FilterDenConstantOutMin=[]  FilterDenConstantOutMax=[]  PCopyOutDataTypeStr=Inherit: Inherit via back propagation  PCopyOutMin=[]  PCopyOutMax=[]  NCopyOutDataTypeStr=Inherit: Inherit via back propagation  NCopyOutMin=[]  NCopyOutMax=[]  IntegratorContinuousStateAttributes=''  IntegratorStateMustResolveToSignalObject=off  IntegratorRTWStateStorageClass=Auto  FilterContinuousStateAttributes=''  FilterStateMustResolveToSignalObject=off  FilterRTWStateStorageClass=Auto  ParallelPVariant=InternalParameters  IdealPVariant=Disabled  IVariant=InternalParameters  DVariant=InternalParameters  IntegratorVariant=Discrete  SatVariant=Enabled  AWVariant=Passthrough  PCopyVariant=Disabled  TRVariant=Disabled  FdbkBlocksVariant=Forward  IdealPFdbkVariant=Disabled  SatFdbkVariant=Disabled  DerivativeFilterVariant=ForwardEulerFilter  NVariant=InternalParameters  NCopyVariant=Disabled  FilterICVariant=InternalICsFilter  IntegratorICVariant=InternalICs  ExternalResetVariant=Disabled  TRSumVariant=Passthrough  SumFdbkVariant=Disabled  SumVariant=Sum_PID  TsampFilterVariant=InternalTs  TsampNgainVariant=Passthrough  TsampIntegralVariant=Passthrough  ExternalSaturationOutDataTypeStr=Inherit: Same as second input
  PID Controller2 : slpidlib/PID Controller  Controller=PID  Form=Parallel  TimeDomain=Discrete-time  UseExternalTs=off  SampleTime=-1  IntegratorMethod=Forward Euler  FilterMethod=Forward Euler  ControllerParametersSource=internal  P=P_High_Speed  I=0  UseKiTs=on  D=0  N=0  UseFilter=on  TunerSelectOption=Transfer Function Based (PID Tuner App)  InitialConditionSource=internal  InitialConditionForIntegrator=0  InitialConditionForFilter=0  DifferentiatorICPrevScaledInput=0  ExternalReset=none  TrackingMode=off  Kt=1  LimitOutput=on  SatLimitsSource=internal  UpperSaturationLimit=MAX_STEERING_ADJUST  LowerSaturationLimit=-MAX_STEERING_ADJUST  LinearizeAsGain=on  AntiWindupMode=none  Kb=1  LimitIntegrator=off  UpperIntegratorSaturationLimit=inf  LowerIntegratorSaturationLimit=-inf  POutMin=[]  POutMax=[]  IOutMin=[]  IOutMax=[]  DOutMin=[]  DOutMax=[]  NOutMin=[]  NOutMax=[]  SumOutMin=[]  SumOutMax=[]  SaturationOutMin=[]  SaturationOutMax=[]  PParamMin=[]  PParamMax=[]  IParamMin=[]  IParamMax=[]  DParamMin=[]  DParamMax=[]  NParamMin=[]  NParamMax=[]  KbParamMin=[]  KbParamMax=[]  KtParamMin=[]  KtParamMax=[]  KbOutMin=[]  KbOutMax=[]  KtOutMin=[]  KtOutMax=[]  IntegratorOutMin=[]  IntegratorOutMax=[]  FilterOutMin=[]  FilterOutMax=[]  SumI1OutMin=[]  SumI1OutMax=[]  SumI2OutMin=[]  SumI2OutMax=[]  SumI3OutMin=[]  SumI3OutMax=[]  SumI4OutMin=[]  SumI4OutMax=[]  SumDOutMin=[]  SumDOutMax=[]  DifferentiatorOutMin=[]  DifferentiatorOutMax=[]  FilterDiffOutCoefMin=[]  FilterDiffOutCoefMax=[]  ReciprocalOutMin=[]  ReciprocalOutMax=[]  SumDenOutMin=[]  SumDenOutMax=[]  SumNumOutMin=[]  SumNumOutMax=[]  DivideOutMin=[]  DivideOutMax=[]  UdiffTsProdOutMin=[]  UdiffTsProdOutMax=[]  NTsProdOutMin=[]  NTsProdOutMax=[]  UintegralTsProdOutMin=[]  UintegralTsProdOutMax=[]  UngainTsProdOutMin=[]  UngainTsProdOutMax=[]  ClampingZeroOutDataTypeStr=Inherit: Inherit via back propagation  ClampingZeroOutMin=[]  ClampingZeroOutMax=[]  FilterDenConstantOutDataTypeStr=Inherit: Inherit via back propagation  FilterDenConstantOutMin=[]  FilterDenConstantOutMax=[]  PCopyOutDataTypeStr=Inherit: Inherit via back propagation  PCopyOutMin=[]  PCopyOutMax=[]  NCopyOutDataTypeStr=Inherit: Inherit via back propagation  NCopyOutMin=[]  NCopyOutMax=[]  IntegratorContinuousStateAttributes=''  IntegratorStateMustResolveToSignalObject=off  IntegratorRTWStateStorageClass=Auto  FilterContinuousStateAttributes=''  FilterStateMustResolveToSignalObject=off  FilterRTWStateStorageClass=Auto  ParallelPVariant=InternalParameters  IdealPVariant=Disabled  IVariant=InternalParameters  DVariant=InternalParameters  IntegratorVariant=Discrete  SatVariant=Enabled  AWVariant=Passthrough  PCopyVariant=Disabled  TRVariant=Disabled  FdbkBlocksVariant=Forward  IdealPFdbkVariant=Disabled  SatFdbkVariant=Disabled  DerivativeFilterVariant=ForwardEulerFilter  NVariant=InternalParameters  NCopyVariant=Disabled  FilterICVariant=InternalICsFilter  IntegratorICVariant=InternalICs  ExternalResetVariant=Disabled  TRSumVariant=Passthrough  SumFdbkVariant=Disabled  SumVariant=Sum_PID  TsampFilterVariant=InternalTs  TsampNgainVariant=Passthrough  TsampIntegralVariant=Passthrough  ExternalSaturationOutDataTypeStr=Inherit: Same as second input
  Product : Product  Inputs=3
  Rate Limiter : RateLimiter  RisingSlewLimit=MAX_DTHETA_DRIVER  FallingSlewLimit=-MAX_DTHETA_DRIVER  SampleTimeMode=inherited
  Saturation Dynamic : simulink/Discontinuities/Saturation Dynamic  OutMin=[]  OutMax=[]  OutDataTypeStr=Inherit: Same as second input  OutDataType=fixdt(1, 16)  OutScaling=2^-10  DoSatur=off
  Saturation2 : Saturate  UpperLimit=CENTER_STEER_ANGLE_MAX  LowerLimit=-CENTER_STEER_ANGLE_MAX
  Sign : Signum
  Sum : Sum  Inputs=|++
  Switch : Switch  Criteria=u2 ~= 0  SaturateOnIntegerOverflow=off  InputSameDT=off
  Switch1 : Switch  Criteria=u2 ~= 0  SaturateOnIntegerOverflow=off  InputSameDT=off
  steering_angle : Outport
  wires:
  Saturation2/1 -> steering_angle/1
  Rate Limiter/1 -> Saturation2/1
  Switch/1 -> Switch1/1
  Controller Information/1 -> Bus Selector/1
  Bus Selector/3 -> Sign/1, Abs/1  "<yaw_ref>"
  Bus Selector/4 -> 1-D Lookup Table/1, 2-D Lookup Table1/2, 2-D Lookup Table2/2  "<v_cog>"
  2-D Lookup Table1/1 -> Min/1
  2-D Lookup Table2/1 -> Min/2
  Min/1 -> Product/3
  Bus Selector/1 -> PID Controller1/1, PID Controller2/1, PID Controller/1  "<p_error>"
  Product/1 -> Sum/2
  Saturation Dynamic/1 -> 2-D Lookup Table1/1, 2-D Lookup Table2/1
  Bus Selector/2 -> GreaterThan/1  "<Vnow>"
  Abs/1 -> Saturation Dynamic/3, Saturation Dynamic/2
  1-D Lookup Table/1 -> Saturation Dynamic/1
  PID Controller/1 -> Switch/3
  PID Controller1/1 -> Switch/1
  Constant/1 -> GreaterThan/2
  Sign/1 -> GreaterThan1/1, Switch/2, Product/2
  Switch1/1 -> Sum/1
  PID Controller2/1 -> Switch1/3
  Constant1/1 -> GreaterThan1/2
  GreaterThan/1 -> NOT/1, NAND/1
  GreaterThan1/1 -> NAND/2
  NAND/1 -> Switch1/2
  NOT/1 -> Product/1
  Sum/1 -> Rate Limiter/1

== system car_model/Driver & Environment/Longitudinal Control ==
  Controller Information : Inport
  In2 : Inport  Port=2
  Sweep Information : Inport  Port=3
  In3 : Inport  Port=4
  AAS : Subsystem
  ABS : Subsystem
      settings: PortSchema="{\"entries\":[{\"content\":{\"sides\":[{\"content\":{\"connectorIds\":[\"In1\",\"In2\",\"In3\"]},\"type\":\"ConnectorPlacement.EquallySpacedRectSide\",\"uuid\":\"05691032-3f39-4834-938a-125b9d9c5bbe\"},{\"content\":{\"connectorIds\":[\"Out1\",\"In5\"],\"side\":\"RIGHT\"},\"type\":\"ConnectorPlacement.EquallySpacedRectSide\",\"uuid\":\"b6342b01-7e0e-4c31-ae65-daa263149cd6\"},{\"content\":{\"connectorIds\":[\"In4\"],\"side\":\"TOP\"},\"type\":\"ConnectorPlacement.EquallySpacedRectSide\",\"uuid\":\"252d477f-1200-4151-9883-b9a128e2c38a\"}]},\"type\":\"ConnectorPlacement.EquallySpacedConnector\",\"uuid\":\"d67aaf26-3760-4411-918f-de910c7b3ed9\"}],\"packageUris\":[\"http://schema.mathworks.com/mf0/Connector/R2020b\"],\"version\":\"1.0\"}"
  Bus Selector : BusSelector  OutputSignals=omega,v_error
  Bus Selector1 : BusSelector  OutputSignals=Velocity Error
  Constant5 : Constant  Value=YAW_ENABLE
  Pedal Positioner : Subsystem
      settings: PortSchema="{\"entries\":[{\"content\":{\"sides\":[{\"content\":{\"connectorIds\":[\"In1\"]},\"type\":\"ConnectorPlacement.EquallySpacedRectSide\",\"uuid\":\"c84d1b45-47cb-44c3-9bb8-057964d890de\"},{\"content\":{\"connectorIds\":[\"Out1\",\"In2\"],\"side\":\"RIGHT\"},\"type\":\"ConnectorPlacement.EquallySpacedRectSide\",\"uuid\":\"136455d0-d36a-4818-af11-72b5a1b8c27c\"},{\"content\":{\"connectorIds\":[],\"side\":\"TOP\"},\"type\":\"ConnectorPlacement.EquallySpacedRectSide\",\"uuid\":\"42b2ce8c-2720-4fbc-908c-f7068b304798\"}]},\"type\":\"ConnectorPlacement.EquallySpacedConnector\",\"uuid\":\"ec27d525-5c9d-4748-8b13-bb528198656f\"}],\"packageUris\":[\"http://schema.mathworks.com/mf0/Connector/R2020b\"],\"version\":\"1.0\"}"
  Switch1 : Switch  Criteria=u2 > Threshold  SaturateOnIntegerOverflow=off  InputSameDT=off
  Unit Delay4 : UnitDelay  SampleTime=-1  HasFrameUpgradeWarning=on
  Unit Delay5 : UnitDelay  SampleTime=-1  HasFrameUpgradeWarning=on
  driver_input : Outport  PortDimensions=1
  brake_pedal : Outport  Port=2
  wires:
  Controller Information/1 -> Bus Selector/1
  Constant5/1 -> Switch1/2
  Sweep Information/1 -> Bus Selector1/1
  Bus Selector1/1 -> Switch1/3  "<Velocity Error>"
  Bus Selector/2 -> Pedal Positioner/1(<v_error>), Switch1/1  "<v_error>"
  Bus Selector/1 -> Unit Delay4/1  "<omega>"
  Switch1/1 -> Unit Delay5/1
  Unit Delay4/1 -> ABS/1(omega)
  Unit Delay5/1 -> ABS/3(<v_error>), AAS/1(v_error)
  AAS/1(driver_input) -> driver_input/1, Pedal Positioner/2(driver_input)
  ABS/1(Px) -> brake_pedal/1
  Pedal Positioner/1(brake) -> ABS/5(ABS_ENABLE)
  In3/1 -> ABS/4(In3)
  In2/1 -> ABS/2(In2)

== system car_model/Driver & Environment/Reference Generator ==
  Analog Signals : Inport
  Driver Information : BusCreator  Inputs=14
  Memory : Memory  InitialCondition=1
  Memory1 : Memory  InitialCondition=1
  Reference Geneator : MATLAB Function  TreatAsAtomicUnit=on  SystemSampleTime=driver_t
  Selector : BusSelector  OutputSignals=psi,Vel,r,Disp,Omega
  Subsystem : Subsystem
  Terminator : Terminator
  Terminator1 : Terminator
  To Workspace : ToWorkspace  VariableName=Driver_Signals  SaveFormat=Timeseries  SampleTime=-1
  To Workspace1 : ToWorkspace  VariableName=Reference_Generator  SaveFormat=Timeseries  SampleTime=-1
  Unit Delay : UnitDelay  SampleTime=-1  HasFrameUpgradeWarning=on
  Unit Delay1 : UnitDelay  InitialCondition=1000  SampleTime=-1  HasFrameUpgradeWarning=on
  Controller Information : Outport
  wires:
  Analog Signals/1 -> To Workspace/1, Selector/1  "Driver"
  Selector/1 -> Subsystem/1(<psi>)  "<psi>"
  Reference Geneator/5(d_error) -> Driver Information/4
  Driver Information/1 -> To Workspace1/1, Controller Information/1  "Driver Information"
  Selector/2 -> Reference Geneator/4(Vg)  "<Vel>"
  Reference Geneator/7(v_error) -> Driver Information/3
  Reference Geneator/8(v_cog) -> Driver Information/6
  Subsystem/1(psi_rev) -> Reference Geneator/3(psi)
  Reference Geneator/6(psi_error) -> Driver Information/5
  Reference Geneator/2(index_all) -> Memory/1, Driver Information/2  "index_all"
  Memory/1 -> Reference Geneator/2("index_all ")
  Reference Geneator/9(r_ref) -> Driver Information/7
  Reference Geneator/10(r_error) -> Driver Information/8
  Reference Geneator/17(ahead) -> Unit Delay/1
  Unit Delay/1 -> Reference Geneator/8("ahead ")
  Reference Geneator/14(omega) -> Driver Information/12
  Reference Geneator/11(x_ref) -> Driver Information/9
  Reference Geneator/12(y_ref) -> Driver Information/10
  Selector/3 -> Reference Geneator/5(yaw)  "<r>"
  Selector/4 -> Reference Geneator/6(pos)  "<Disp>"
  Reference Geneator/13(yaw_ref) -> Driver Information/11
  Memory1/1 -> Reference Geneator/1("index_small ")
  Reference Geneator/18(di_now) -> Unit Delay1/1
  Unit Delay1/1 -> Reference Geneator/9(di_prev)
  Selector/5 -> Reference Geneator/7("omega ")  "<Omega>"
  Reference Geneator/15(p_error) -> Driver Information/13
  Reference Geneator/16(Vnow) -> Driver Information/14
  Reference Geneator/4(index_small) -> Memory1/1, Driver Information/1  "index_small"
  Reference Geneator/1(sign_distance) -> Terminator/1
  Reference Geneator/3(min_d) -> Terminator1/1

== system car_model/Driver & Environment/Sweep Generator ==
  Analog Signals : Inport
  Bus Creator : BusCreator  Inputs=2
  Bus Selector : BusSelector  OutputSignals=Vel
  Memory : Memory  InitialCondition=1
  Sweep Generator : MATLAB Function  TreatAsAtomicUnit=on  SystemSampleTime=driver_t
  To Workspace : ToWorkspace  VariableName=counter  SaveFormat=Timeseries  SampleTime=-1
  Unit Delay : UnitDelay  SampleTime=-1  HasFrameUpgradeWarning=on
  Unit Delay1 : UnitDelay  InitialCondition=1  SampleTime=-1  HasFrameUpgradeWarning=on
  Controller Information : Outport
  wires:
  Analog Signals/1 -> Bus Selector/1
  Sweep Generator/2(vel_err) -> Bus Creator/1  "Velocity Error"
  Sweep Generator/3(ref_steer) -> Bus Creator/2  "Steering Angle"
  Bus Creator/1 -> Controller Information/1
  Bus Selector/1 -> Sweep Generator/2(vel)  "<Vel>"
  Sweep Generator/1(index) -> Memory/1
  Memory/1 -> Sweep Generator/1("index ")
  Sweep Generator/5(counter) -> Unit Delay/1, To Workspace/1
  Unit Delay/1 -> Sweep Generator/4("counter ")
  Sweep Generator/4(ON) -> Unit Delay1/1
  Unit Delay1/1 -> Sweep Generator/3("ON ")

== system car_model/Vehicle Model/Electronics ==
  Veh : Inport
  Sus : Inport  Port=2
  Whl : Inport  Port=3
  Trn : Inport  Port=4
  All Veh Info : BusCreator  Inputs=veh,sus,whl,trn
  Bus Selector2 : BusSelector  OutputSignals=veh.InertFrm.Cg.Disp,veh.InertFrm.Cg.Ang.psi,veh.BdyFrm.Cg.Vel,veh.BdyFrm.Cg.AngVel.r,sus.Sus.steering_angle,whl.TireFrame.Omega,whl.TireFrame.GndFz  OutputAsBus=on
  Cooling Sensors : Subsystem
  Corner Dynamics Sensors : Subsystem
  Digital SIgnals : BusCreator  Inputs=4
  Navigation Sensors : Subsystem
  Power Sensors : Subsystem
  To Workspace : ToWorkspace  VariableName=Digital_Signals  SaveFormat=Timeseries  SampleTime=-1
  To Workspace1 : ToWorkspace  VariableName=Vehicle_Signals  SaveFormat=Timeseries  SampleTime=-1
  Analog Signals : Outport
  Digital Signals : Outport  Port=2
  wires:
  Sus/1 -> All Veh Info/2
  Whl/1 -> All Veh Info/3
  Veh/1 -> All Veh Info/1
  Trn/1 -> All Veh Info/4
  Bus Selector2/1 -> Analog Signals/1
  Navigation Sensors/1(Navigation Sensors) -> Digital SIgnals/1  "Navigation Sensors"
  Power Sensors/1(Power Sensors) -> Digital SIgnals/2  "Power Sensors"
  Corner Dynamics Sensors/1(Corner Dynamics Sensors) -> Digital SIgnals/4  "Corner Dynamics Sensors"
  Digital SIgnals/1 -> Digital Signals/1, To Workspace/1  "Digital Signls"
  Cooling Sensors/1(Cooling Sensors) -> Digital SIgnals/3  "Cooling Sensors"
  All Veh Info/1 -> Bus Selector2/1, To Workspace1/1, Navigation Sensors/1(Analog Signals), Corner Dynamics Sensors/1(Analog Signals), Cooling Sensors/1(Analog Signals), Power Sensors/1(Analog Signals)
